simulink model "joint_control_calibration_v1"  (R2016a)
settings: Solver=FixedStepDiscrete  StartTime=0.0  StopTime=inf  FixedStep=0.001  RelTol=1e-3
undefined symbols (not defined in the file or in its folder): Left_Leg
libraries: xpcethercatlib x7, slrtlib x4, simulink x3
settings Model: xpc_rtwmakecfg_data=_xpcethercatlib_  SimulationMode=external  Creator=Projectmarch  LastModifiedBy=Projectmarch
settings SolverCC: EnableConcurrentExecution=on
settings DataIOCC: SaveFormat=StructureWithTime
settings OptimizationCC: BlockReduction=off  OptimizeBlockIOStorage=off  BufferReuse=off  GlobalBufferReuse=off  ExpressionFolding=off  LocalBlockOutputs=off
settings HardwareCC: ProdBitPerPointer=32  ProdLargestAtomicFloat=None  ProdWordSize=32  ProdLongLongMode=on  ProdHWDeviceType=Generic->32-bit x86 compatible
settings RTWCC: SystemTargetFile=slrt.tlc  TemplateMakefile=slrt_default_tmf  Description=Simulink Real-Time  RTWCompilerOptimization=on

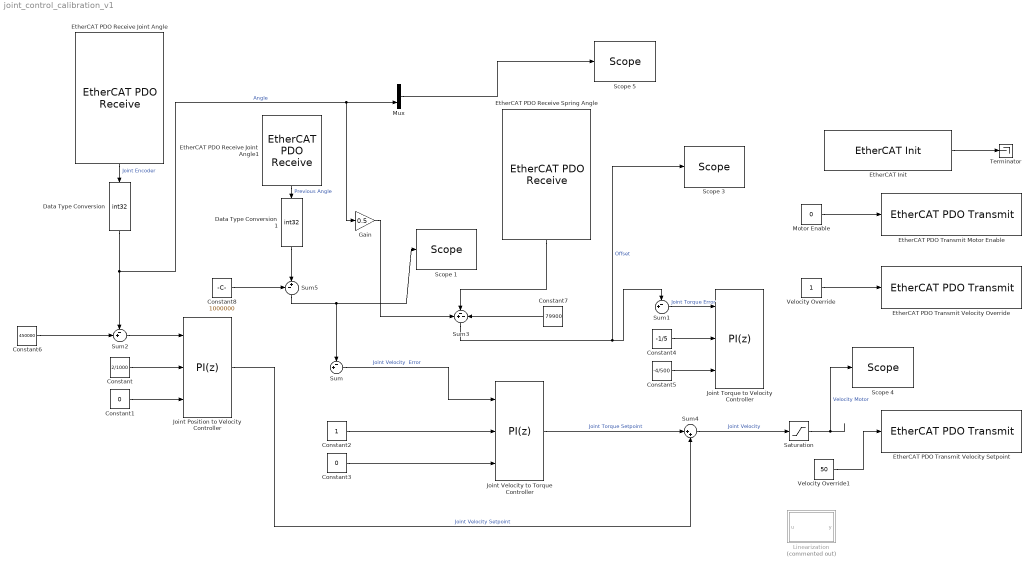
== system joint_control_calibration_v1 ==
  Constant : Constant  Value=2/1000
  Constant1 : Constant  Value=0
  Constant2 : Constant
  Constant3 : Constant  Value=0
  Constant4 : Constant  Value=-1/5
  Constant5 : Constant  Value=-4/500
  Constant6 : Constant  Value=450000
  Constant7 : Constant  Value=79900
  Constant8 : Constant  Value=1000000
  Data Type Conversion : DataTypeConversion  OutDataTypeStr=int32
  Data Type Conversion1 : DataTypeConversion  OutDataTypeStr=int32
  "EtherCAT Init " : xpcethercatlib/EtherCAT Init   Priority=0  config_file=D:\Software\MATLAB\simulink-models\EtherCAT Config files\full_setup_v1.0.xml  device_id=0  pci_bus=2  pci_slot=0  dctuning=2  enaDebug=off  enaDC=on  errLink=off  masterDbg=off  stateChgDbg=off  baseClock=off  masterCfg=off  logFile='c:\dbglog.txt'  sample_time=0.001000
  EtherCAT PDO Receive Joint Angle : xpcethercatlib/EtherCAT PDO Receive  Priority=2  sig_name=Left_Leg.Inputs.H_jointAngle  sig_offset=1144  sig_type=uint32  type_size=32  sig_dim=1  device_id=0  sample_time=0.001000
  EtherCAT PDO Receive Joint Angle1 : xpcethercatlib/EtherCAT PDO Receive  Priority=2  sig_name=Left_Leg.Inputs.K_footForceFront[0]  sig_offset=1464  sig_type=int32  type_size=32  sig_dim=1  device_id=0  sample_time=0.001000
  EtherCAT PDO Receive Spring Angle : xpcethercatlib/EtherCAT PDO Receive  Priority=2  sig_name=Left_Leg.Inputs.H_springAngle  sig_offset=1176  sig_type=uint32  type_size=32  sig_dim=1  device_id=0  sample_time=0.001000
  EtherCAT PDO Transmit Motor Enable : xpcethercatlib/EtherCAT PDO Transmit   Priority=3  sig_name=Left_Leg.Outputs.H_motorEnable  sig_offset=1192  sig_type=uint8  type_size=8  sig_dim=1  device_id=0  sample_time=0.001000
  EtherCAT PDO Transmit Velocity Override : xpcethercatlib/EtherCAT PDO Transmit   Priority=3  sig_name=Left_Leg.Outputs.H_data[4]  sig_offset=1400  sig_type=int32  type_size=32  sig_dim=1  device_id=0  sample_time=0.001000
  "EtherCAT PDO Transmit Velocity Setpoint " : xpcethercatlib/EtherCAT PDO Transmit   Priority=3  sig_name=Left_Leg.Outputs.H_velocitySetPoint  sig_offset=1144  sig_type=int16  type_size=16  sig_dim=1  device_id=0  sample_time=0.001000
  Gain : Gain  Gain=0.5
  Joint Position to Velocity Controller : simulink/Continuous/PID Controller  Controller=PI  TimeDomain=Discrete-time  SampleTime=0.001  IntegratorMethod=Forward Euler  FilterMethod=Forward Euler  Form=Parallel  UseFilter=off  ControllerParametersSource=external  P=1  I=1  D=0  N=100  InitialConditionSource=internal  InitialConditionForIntegrator=0  InitialConditionForFilter=0  ExternalReset=none  LimitOutput=off  UpperSaturationLimit=inf  LowerSaturationLimit=-inf  LinearizeAsGain=off  AntiWindupMode=none  Kb=1  TrackingMode=off  Kt=1  PParamMin=[]  PParamMax=[]  IParamMin=[]  IParamMax=[]  DParamMin=[]  DParamMax=[]  NParamMin=[]  NParamMax=[]  KbParamMin=[]  KbParamMax=[]  KtParamMin=[]  KtParamMax=[]  POutMin=[]  POutMax=[]  IOutMin=[]  IOutMax=[]  DOutMin=[]  DOutMax=[]  NOutMin=[]  NOutMax=[]  KbOutMin=[]  KbOutMax=[]  KtOutMin=[]  KtOutMax=[]  IntegratorOutMin=[]  IntegratorOutMax=[]  FilterOutMin=[]  FilterOutMax=[]  SumOutMin=[]  SumOutMax=[]  SumI1OutMin=[]  SumI1OutMax=[]  SumI2OutMin=[]  SumI2OutMax=[]  SumI3OutMin=[]  SumI3OutMax=[]  SumDOutMin=[]  SumDOutMax=[]  SaturationOutMin=[]  SaturationOutMax=[]  IntegratorContinuousStateAttributes=''  IntegratorStateMustResolveToSignalObject=off  IntegratorRTWStateStorageClass=Auto  FilterContinuousStateAttributes=''  FilterStateMustResolveToSignalObject=off  FilterRTWStateStorageClass=Auto  DifferentiatorICPrevScaledInput=0  DifferentiatorOutMin=[]  DifferentiatorOutMax=[]
  Joint Torque to Velocity Controller : simulink/Continuous/PID Controller  Controller=PI  TimeDomain=Discrete-time  SampleTime=0.001  IntegratorMethod=Forward Euler  FilterMethod=Forward Euler  Form=Parallel  UseFilter=off  ControllerParametersSource=external  P=1  I=1  D=0  N=100  InitialConditionSource=internal  InitialConditionForIntegrator=0  InitialConditionForFilter=0  ExternalReset=none  LimitOutput=off  UpperSaturationLimit=inf  LowerSaturationLimit=-inf  LinearizeAsGain=off  AntiWindupMode=none  Kb=1  TrackingMode=off  Kt=1  PParamMin=[]  PParamMax=[]  IParamMin=[]  IParamMax=[]  DParamMin=[]  DParamMax=[]  NParamMin=[]  NParamMax=[]  KbParamMin=[]  KbParamMax=[]  KtParamMin=[]  KtParamMax=[]  POutMin=[]  POutMax=[]  IOutMin=[]  IOutMax=[]  DOutMin=[]  DOutMax=[]  NOutMin=[]  NOutMax=[]  KbOutMin=[]  KbOutMax=[]  KtOutMin=[]  KtOutMax=[]  IntegratorOutMin=[]  IntegratorOutMax=[]  FilterOutMin=[]  FilterOutMax=[]  SumOutMin=[]  SumOutMax=[]  SumOutDataTypeStr=double  SumI1OutMin=[]  SumI1OutMax=[]  SumI2OutMin=[]  SumI2OutMax=[]  SumI3OutMin=[]  SumI3OutMax=[]  SumDOutMin=[]  SumDOutMax=[]  SaturationOutMin=[]  SaturationOutMax=[]  IntegratorContinuousStateAttributes=''  IntegratorStateMustResolveToSignalObject=off  IntegratorRTWStateStorageClass=Auto  FilterContinuousStateAttributes=''  FilterStateMustResolveToSignalObject=off  FilterRTWStateStorageClass=Auto  DifferentiatorICPrevScaledInput=0  DifferentiatorOutMin=[]  DifferentiatorOutMax=[]
  Joint Velocity to Torque Controller : simulink/Continuous/PID Controller  Controller=PI  TimeDomain=Discrete-time  SampleTime=0.001  IntegratorMethod=Forward Euler  FilterMethod=Forward Euler  Form=Parallel  UseFilter=off  ControllerParametersSource=external  P=1  I=1  D=0  N=100  InitialConditionSource=internal  InitialConditionForIntegrator=0  InitialConditionForFilter=0  ExternalReset=none  LimitOutput=off  UpperSaturationLimit=inf  LowerSaturationLimit=-inf  LinearizeAsGain=off  AntiWindupMode=none  Kb=1  TrackingMode=off  Kt=1  PParamMin=[]  PParamMax=[]  IParamMin=[]  IParamMax=[]  DParamMin=[]  DParamMax=[]  NParamMin=[]  NParamMax=[]  KbParamMin=[]  KbParamMax=[]  KtParamMin=[]  KtParamMax=[]  POutMin=[]  POutMax=[]  IOutMin=[]  IOutMax=[]  DOutMin=[]  DOutMax=[]  NOutMin=[]  NOutMax=[]  KbOutMin=[]  KbOutMax=[]  KtOutMin=[]  KtOutMax=[]  IntegratorOutMin=[]  IntegratorOutMax=[]  FilterOutMin=[]  FilterOutMax=[]  SumOutMin=[]  SumOutMax=[]  SumI1OutMin=[]  SumI1OutMax=[]  SumI2OutMin=[]  SumI2OutMax=[]  SumI3OutMin=[]  SumI3OutMax=[]  SumDOutMin=[]  SumDOutMax=[]  SaturationOutMin=[]  SaturationOutMax=[]  IntegratorContinuousStateAttributes=''  IntegratorStateMustResolveToSignalObject=off  IntegratorRTWStateStorageClass=Auto  FilterContinuousStateAttributes=''  FilterStateMustResolveToSignalObject=off  FilterRTWStateStorageClass=Auto  DifferentiatorICPrevScaledInput=0  DifferentiatorOutMin=[]  DifferentiatorOutMax=[]
  Linearization : MATLAB Function  Commented=on  TreatAsAtomicUnit=on
  Motor Enable : Constant  Value=0  OutDataTypeStr=uint8
  Mux : Mux  Inputs=2
  Saturation : Saturate  UpperLimit=200  LowerLimit=-200
  Scope 1 : slrtlib/Displays and Logging/Scope   scopeno=2  scopetype=Target  autostart=on  viewmode=Graphical sliding  formatstr='%15.6f'  grid=on  ylimits=[0,0]  nosamples=10000  noprepostsamples=0  interleave=1  triggermode=FreeRun  triggersignal=1  trigsignalfromport=off  triggerlevel=0.0  triggerslope=Either  triggerscope=1  triggersample=0  filename=data.dat  mode=Lazy  writesize=512  autorestart=off  dynamicfilemode=off  maxwritefilesize=512*1024^2
  Scope 3 : slrtlib/Displays and Logging/Scope   scopeno=3  scopetype=Target  autostart=on  viewmode=Graphical sliding  formatstr='%15.6f'  grid=on  ylimits=[0,0]  nosamples=10000  noprepostsamples=0  interleave=1  triggermode=FreeRun  triggersignal=1  trigsignalfromport=off  triggerlevel=0.0  triggerslope=Either  triggerscope=1  triggersample=0  filename=data.dat  mode=Lazy  writesize=512  autorestart=off  dynamicfilemode=off  maxwritefilesize=512*1024^2
  Scope 4 : slrtlib/Displays and Logging/Scope   scopeno=4  scopetype=Target  autostart=on  viewmode=Graphical sliding  formatstr='%15.6f'  grid=on  ylimits=[0,0]  nosamples=10000  noprepostsamples=0  interleave=1  triggermode=FreeRun  triggersignal=1  trigsignalfromport=off  triggerlevel=0.0  triggerslope=Either  triggerscope=1  triggersample=0  filename=data.dat  mode=Lazy  writesize=512  autorestart=off  dynamicfilemode=off  maxwritefilesize=512*1024^2
  Scope 5 : slrtlib/Displays and Logging/Scope   scopeno=1  scopetype=Target  autostart=on  viewmode=Graphical sliding  formatstr='%15.6f'  grid=on  ylimits=[0,0]  nosamples=10000  noprepostsamples=0  interleave=1  triggermode=FreeRun  triggersignal=1  trigsignalfromport=off  triggerlevel=0.0  triggerslope=Either  triggerscope=1  triggersample=0  filename=data.dat  mode=Lazy  writesize=512  autorestart=off  dynamicfilemode=off  maxwritefilesize=512*1024^2
  Sum{,1..2,5} (4 alike) : Sum  Inputs=-+|
  Sum3 : Sum  Inputs=+--
  Sum4 : Sum  Inputs=|++  OutDataTypeStr=int16
  Terminator : Terminator
  Velocity Override : Constant  OutDataTypeStr=int32
  Velocity Override1 : Constant  Value=50  OutDataTypeStr=int16
  wires:
  Joint Velocity to Torque Controller/1 -> Sum4/1  "Joint Torque Setpoint"
  Joint Position to Velocity Controller/1 -> Sum4/2  "Joint Velocity Setpoint"
  Sum/1 -> Joint Velocity to Torque Controller/1  "Joint Velocity  Error"
  Constant/1 -> Joint Position to Velocity Controller/2
  Constant1/1 -> Joint Position to Velocity Controller/3
  Constant2/1 -> Joint Velocity to Torque Controller/2
  Constant3/1 -> Joint Velocity to Torque Controller/3
  Constant4/1 -> Joint Torque to Velocity Controller/2
  Constant5/1 -> Joint Torque to Velocity Controller/3
  Sum2/1 -> Joint Position to Velocity Controller/1
  Constant6/1 -> Sum2/2
  "EtherCAT Init "/1 -> Terminator/1
  Velocity Override/1 -> EtherCAT PDO Transmit Velocity Override/1
  Motor Enable/1 -> EtherCAT PDO Transmit Motor Enable/1
  EtherCAT PDO Receive Spring Angle/1 -> Sum3/2
  Sum3/1 -> Scope 3/1, Sum1/1  "Offset"
  Sum4/1 -> Saturation/1  "Joint Velocity"
  Gain/1 -> Sum3/1
  Constant7/1 -> Sum3/3
  Saturation/1 -> Scope 4/1  "Velocity Motor"
  EtherCAT PDO Receive Joint Angle1/1 -> Data Type Conversion1/1  "Previous Angle"
  EtherCAT PDO Receive Joint Angle/1 -> Data Type Conversion/1  "Joint Encoder"
  Data Type Conversion/1 -> Gain/1, Mux/2, Sum2/1  "Angle"
  Mux/1 -> Scope 5/1
  Data Type Conversion1/1 -> Sum5/2
  Sum5/1 -> Sum/1, Scope 1/1
  Constant8/1 -> Sum5/1
  Sum1/1 -> Joint Torque to Velocity Controller/1  "Joint Torque Error"
  Velocity Override1/1 -> "EtherCAT PDO Transmit Velocity Setpoint "/1

== matlab function joint_control_calibration_v1/Linearization ==
  data: u input; y output
function y = fcn(u)
%#codegen
rd = 44.8/1000;
L0 = 75.98/1000;
rp = 105.658/1000;

angleRad = LKFE_jointMin + (LKFE_jointMax-LKFE_jointMin)/(LKFE_encMax-LKFE_encMin)*(encoderValue-LKFE_encMin);

offsetAngle = 3.14 - acos((L0^2 - rp^2 - rd^2)/(-2*rp*rd));

angleCorrected = angle - offsetAngle;

l = sqrt(rp^2 + rd^2 + 2*rp*rd*cos(angleCorrected));
d = rp*rd*sin(-angleCorrected)/l;

N = rd/d;


y = N*u;
